simulink model "dq0_fun3"  (R2020b)
settings: Solver=FixedStepAuto  StartTime=0.0  StopTime=tStop  FixedStep=tStep  RelTol=1e-3
values from neighbouring files (symbols this model uses):
  amp = [0, amplitude]    [dq_new.m]    (also in dq_small.m = [0, 1]; dq_test.m)
  f_c = 50    [dq_new.m]    (also in dq_small.m; dq_test.m)
  freq = [f_meas f_meas]    [dq_new.m]    (also in dq_small.m = [f_p f_p]; dq_test.m = [freq_meas(1,i) freq_meas(1,i)]; test1.m = logspace(-2,4,20))
  L = 27e-3    (= 0.027)    [dq_new.m]    (also in dq_small.m; dq_test.m; script.m = 1; untitled.m = 1500)
  R = 15    [dq_new.m]    (also in dq_small.m; dq_test.m; script.m = 10)
libraries: powerlib x16, powerlib_meascontrol x7
settings Model: Creator=kacper  LastModifiedBy=kacper

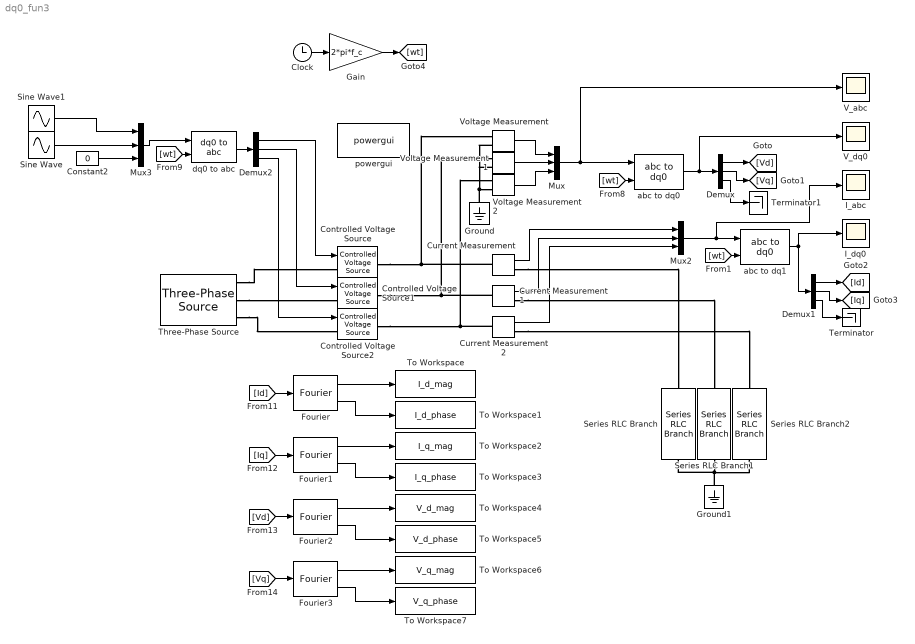
== system dq0_fun3 ==
  Clock : Clock
  Constant2 : Constant  Value=0
  Controlled Voltage Source : powerlib/Electrical Sources/Controlled Voltage Source  Initialize=on  Source_Type=AC  Amplitude=0  Phase=0  Frequency=0  Measurements=None
  Controlled Voltage Source1 : powerlib/Electrical Sources/Controlled Voltage Source  Initialize=on  Source_Type=AC  Amplitude=0  Phase=0  Frequency=0  Measurements=None
  Controlled Voltage Source2 : powerlib/Electrical Sources/Controlled Voltage Source  Initialize=on  Source_Type=AC  Amplitude=0  Phase=0  Frequency=0  Measurements=None
  Current Measurement : powerlib/Measurements/Current Measurement  PhasorSimulation=off  OutputType=Complex  PSBequivalent=0
  Current Measurement1 : powerlib/Measurements/Current Measurement  PhasorSimulation=off  OutputType=Complex  PSBequivalent=0
  Current Measurement2 : powerlib/Measurements/Current Measurement  PhasorSimulation=off  OutputType=Complex  PSBequivalent=0
  Demux : Demux  Outputs=3
  Demux1 : Demux  Outputs=3
  Demux2 : Demux  Outputs=3
  Fourier{,1..3} (4 alike) : powerlib_meascontrol/Measurements/Fourier  Freq=freq(1,1)  n=1  InInit=[0, 90]  Ts=0
  Gain : Gain  Gain=2*pi*f_c
  Ground : powerlib/Elements/Ground  LConnTagsString=a
  Ground1 : powerlib/Elements/Ground  LConnTagsString=a
  I_abc : Scope
  I_dq0 : Scope
  Mux : Mux  Inputs=3
  Mux2 : Mux  Inputs=3
  Mux3 : Mux  Inputs=3
  Series RLC Branch : powerlib/Elements/Series RLC Branch  LConnTagsString=__new0  RConnTagsString=__new0  BranchType=RL  Resistance=R  Inductance=L  SetiL0=off  InitialCurrent=0  Capacitance=1e-6  Setx0=off  InitialVoltage=0  Measurements=None
  Series RLC Branch1 : powerlib/Elements/Series RLC Branch  LConnTagsString=__new0  RConnTagsString=__new0  BranchType=RL  Resistance=R  Inductance=L  SetiL0=off  InitialCurrent=0  Capacitance=1e-6  Setx0=off  InitialVoltage=0  Measurements=None
  Series RLC Branch2 : powerlib/Elements/Series RLC Branch  LConnTagsString=__new0  RConnTagsString=__new0  BranchType=RL  Resistance=R  Inductance=L  SetiL0=off  InitialCurrent=0  Capacitance=1e-6  Setx0=off  InitialVoltage=0  Measurements=None
  Sine Wave : Sin  Amplitude=amp(1,2)  Frequency=2*pi*freq(1,2)  SampleTime=0
  Sine Wave1 : Sin  Amplitude=amp(1,1)  Frequency=2*pi*freq(1,1)  SampleTime=0
  Terminator : Terminator
  Terminator1 : Terminator
  Three-Phase Source : powerlib/Electrical Sources/Three-Phase Source  InternalConnection=Yg  VoltagePhases=off  Voltage=0  PhaseAngle=0  Voltage_phases=[25e3 25e3 25e3]/sqrt(3)  PhaseAngles_phases=[0 -120 +120]  Frequency=f_c  NonIdealSource=off  SpecifyImpedance=off  Resistance=0.8929  Inductance=16.58e-3  ShortCircuitLevel=100e6  BaseVoltage=25e3  XRratio=7  BusType=swing  Pref=10e3  Qref=0  Prefabc=[10e3, 10e3, 10e3]  Qrefabc=[0, 0, 0]  Qmin=-inf  Qmax=inf
  To Workspace : ToWorkspace  VariableName=I_d_mag  SampleTime=-1
  To Workspace1 : ToWorkspace  VariableName=I_d_phase  SampleTime=-1
  To Workspace2 : ToWorkspace  VariableName=I_q_mag  SampleTime=-1
  To Workspace3 : ToWorkspace  VariableName=I_q_phase  SampleTime=-1
  To Workspace4 : ToWorkspace  VariableName=V_d_mag  SampleTime=-1
  To Workspace5 : ToWorkspace  VariableName=V_d_phase  SampleTime=-1
  To Workspace6 : ToWorkspace  VariableName=V_q_mag  SampleTime=-1
  To Workspace7 : ToWorkspace  VariableName=V_q_phase  SampleTime=-1
  V_abc : Scope
  V_dq0 : Scope
  Voltage Measurement : powerlib/Measurements/Voltage Measurement  PhasorSimulation=off  OutputType=Complex  PSBequivalent=0
  Voltage Measurement1 : powerlib/Measurements/Voltage Measurement  PhasorSimulation=off  OutputType=Complex  PSBequivalent=0
  Voltage Measurement2 : powerlib/Measurements/Voltage Measurement  PhasorSimulation=off  OutputType=Complex  PSBequivalent=0
  abc to dq0 : powerlib_meascontrol/Transformations/abc to dq0  Alignment=90 degrees behind phase A axis
  abc to dq1 : powerlib_meascontrol/Transformations/abc to dq0  Alignment=90 degrees behind phase A axis
  dq0 to abc : powerlib_meascontrol/Transformations/dq0 to abc  Alignment=90 degrees behind phase A axis
  powergui : powerlib/powergui  Priority=1  SimulationMode=Continuous  SampleTime=50e-6  frequency=60  Iterations=50  frequencyindice=0  Pbase=100e6  ErrMax=1e-4  UnitsV=kV  UnitsW=MW  buscounter=0  FunctionMessages=off  echomessages=off  EnableUseOfTLC=off  CurrentSourceSwitches=off  DisableSnubberDevices=off  DisableRonSwitches=off  DisableVfSwitches=off  DisplayEquations=off  AutomaticDiscreteSolvers=off  SolverType=Tustin/Backward Euler (TBE)  Interpol=off  ExternalGateDelay=off  methode=off  Ts=100  x0status=blocks  SPID=on  SwTol=0  HookPort=off  NonlinearTolerance=1e-4  nMaxIteration=100  ContinueOnMaxIteration=off  RestoreLinks=warning  ResistiveCurrentMeasurement=off  Frange=[0:2:500]  Ylog=off  Xlog=on  ShowGrid=off  save=off  variable=ZData  structure=0  ZoomFFT=off  StartTime=0.0  cycles=1  DisplayStyle=1  fundamental=60  FreqAxis=off  MaxFrequency=1000  frequencyindicesteady=1  RmsSteady=1  display=off
  wires:
  Voltage Measurement1/1 -> Mux/2
  Voltage Measurement/1 -> Mux/1
  Voltage Measurement2/1 -> Mux/3
  Mux/1 -> V_abc/1, abc to dq0/1
  abc to dq0/1 -> Demux/1, V_dq0/1
  Current Measurement/1 -> Mux2/1
  Current Measurement1/1 -> Mux2/2
  Current Measurement2/1 -> Mux2/3
  Mux2/1 -> I_abc/1, abc to dq1/1
  abc to dq1/1 -> I_dq0/1, Demux1/1
  Demux/1 -> [Vd]
  Demux/2 -> [Vq]
  Demux1/1 -> [Id]
  Demux1/2 -> [Iq]
  dq0 to abc/1 -> Demux2/1
  Clock/1 -> Gain/1
  Gain/1 -> [wt]
  [wt] -> dq0 to abc/2
  Mux3/1 -> dq0 to abc/1
  Sine Wave1/1 -> Mux3/1
  Sine Wave/1 -> Mux3/2
  Constant2/1 -> Mux3/3
  Demux2/1 -> Controlled Voltage Source/1
  Demux2/2 -> Controlled Voltage Source1/1
  Demux2/3 -> Controlled Voltage Source2/1
  Fourier/1 -> To Workspace/1
  Fourier/2 -> To Workspace1/1
  Fourier1/2 -> To Workspace3/1
  Fourier1/1 -> To Workspace2/1
  Fourier2/2 -> To Workspace5/1
  Fourier2/1 -> To Workspace4/1
  Fourier3/2 -> To Workspace7/1
  Fourier3/1 -> To Workspace6/1
  [Id] -> Fourier/1
  [Iq] -> Fourier1/1
  [Vd] -> Fourier2/1
  [Vq] -> Fourier3/1
  Demux1/3 -> Terminator/1
  Demux/3 -> Terminator1/1
  [wt] -> abc to dq0/2
  [wt] -> abc to dq1/2
  connections:
  Current Measurement/LConn1 -- Controlled Voltage Source/RConn1 -- Voltage Measurement/LConn1
  Current Measurement1/LConn1 -- Controlled Voltage Source1/RConn1 -- Voltage Measurement1/LConn1
  Current Measurement2/LConn1 -- Controlled Voltage Source2/RConn1 -- Voltage Measurement2/LConn1
  Ground/LConn1 -- Voltage Measurement/LConn2 -- Voltage Measurement1/LConn2 -- Voltage Measurement2/LConn2
  Ground1/LConn1 -- Series RLC Branch1/RConn1 -- Series RLC Branch2/RConn1 -- Series RLC Branch/RConn1
  Current Measurement/RConn1 -- Series RLC Branch/LConn1
  Current Measurement1/RConn1 -- Series RLC Branch1/LConn1
  Current Measurement2/RConn1 -- Series RLC Branch2/LConn1
  Three-Phase Source/RConn1 -- Controlled Voltage Source/LConn1
  Three-Phase Source/RConn2 -- Controlled Voltage Source1/LConn1
  Three-Phase Source/RConn3 -- Controlled Voltage Source2/LConn1
